simulink model "part2_1"  (R2021b)
settings: Solver=VariableStepAuto  StartTime=0.0  StopTime=10.0  RelTol=1e-3
undefined symbols (not defined in the file or in its folder): B, s, X, Y
libraries: visiontextngfix x2
settings Model: Creator=setarehdehghanfard  LastModifiedBy=setarehdehghanfard

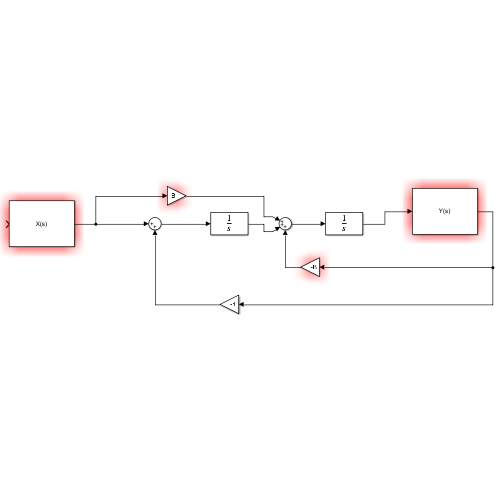
[thumbnail: Simulink's stored preview of the top-level diagram]
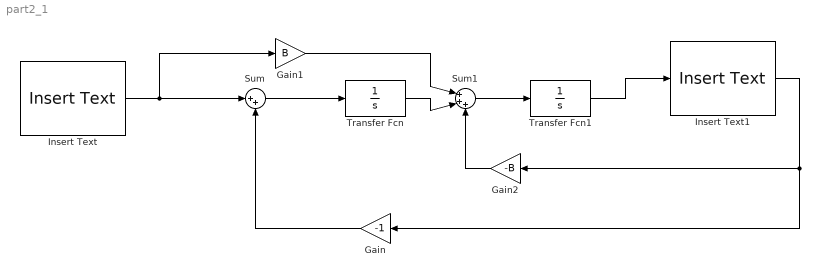
== system part2_1 ==
  Gain : Gain  Gain=-1
  Gain1 : Gain  Gain=B
  Gain2 : Gain  Gain=-B
  Insert Text : visiontextngfix/Insert Text  inputType=Obsolete  theText=X(s)  getTextLocFrom=Specify via dialog  textLoc=[1 1]  getTextColorFrom=Specify via dialog  textColor=[0 0 0]  getTextIntensityFrom=Specify via dialog  textIntensity=0  getTextOpacityFrom=Specify via dialog  textOpacity=1.0  dummyVar2=0  dummyVar3=0  dummyVar4=0  imagePorts=One multidimensional signal  isInputTransposed=off  fontFace=LucidaSansRegular  dummyVar1=0  blockFontSize=12  antiAliased=on
      settings: SourceProductBaseCode=VP
  Insert Text1 : visiontextngfix/Insert Text  inputType=Obsolete  theText=Y(s)  getTextLocFrom=Specify via dialog  textLoc=[1 1]  getTextColorFrom=Specify via dialog  textColor=[0 0 0]  getTextIntensityFrom=Specify via dialog  textIntensity=0  getTextOpacityFrom=Specify via dialog  textOpacity=1.0  dummyVar2=0  dummyVar3=0  dummyVar4=0  imagePorts=One multidimensional signal  isInputTransposed=off  fontFace=LucidaSansRegular  dummyVar1=0  blockFontSize=12  antiAliased=on
      settings: SourceProductBaseCode=VP
  Sum : Sum  Inputs=|++
  Sum1 : Sum  Inputs=|+++
  Transfer Fcn : TransferFcn  Denominator=[1 0]
  Transfer Fcn1 : TransferFcn  Denominator=[1 0]
  wires:
  Gain/1 -> Sum/2
  Sum/1 -> Transfer Fcn/1
  Sum1/1 -> Transfer Fcn1/1
  Gain2/1 -> Sum1/3
  Transfer Fcn/1 -> Sum1/2
  Gain1/1 -> Sum1/1
  Insert Text/1 -> Gain1/1, Sum/1
  Transfer Fcn1/1 -> Insert Text1/1
  Insert Text1/1 -> Gain/1, Gain2/1
